simulink model "model"  (R2022a)
settings: Solver=VariableStepAuto  StartTime=0.0  StopTime=5  RelTol=1e-3  EnableMultiTasking=on
values from neighbouring files (symbols this model uses):
  Ce = 0.556    [Untitled.m]    (also in liner.m)
  Ki = 5    [Untitled.m]    (also in liner.m = 1)
  Kn = 7.84    [Untitled.m]    (also in liner.m = 29.75)
  Ks = 1    [Untitled.m]    (also in liner.m)
  R = 0.6    [Untitled.m]    (also in liner.m)
  Tl = 0.167    [Untitled.m]    (also in liner.m)
  Tm = 0.282    [Untitled.m]    (also in liner.m)
  Toi = 0.0025    [Untitled.m]
  Ton = 0.1    [Untitled.m]
  Ts = 0.01    [Untitled.m]    (also in liner.m)
undefined symbols (not defined in the file or in its folder): alpha, beta, Id, IdN, taui, taun, Ud, UN, Un, Uoil, Uonl
settings Model: Creator=houtonglei  LastModifiedBy=houtonglei
settings SolverCC: AllowMultiTaskInputOutput=on  ConcurrentTasks=on  AlgebraicLoopSolver=TrustRegion  PositivePriorityOrder=on  AutoInsertRateTranBlk=on
settings DataIOCC: SaveFinalState=on
settings OptimizationCC: UseDivisionForNetSlopeComputation=UseDivisionForReciprocalsOfIntegersOnly  GainParamInheritBuiltInType=on  UseFloatMulNetSlope=on  InheritOutputTypeSmallerThanSingle=on  UseRowMajorAlgorithm=on
settings DebuggingCC: ReadBeforeWriteMsg=DisableAll  WriteAfterWriteMsg=DisableAll  WriteAfterReadMsg=DisableAll
settings ModelReferenceCC: EnableParallelModelReferenceBuilds=on  ParallelModelReferenceMATLABWorkerInit=Load Top Model  ModelReferenceMinAlgLoopOccurrences=on
settings SFSimCC: SFSimEcho=off  CustomCodeUndefinedFunction=UseInterfaceOnly

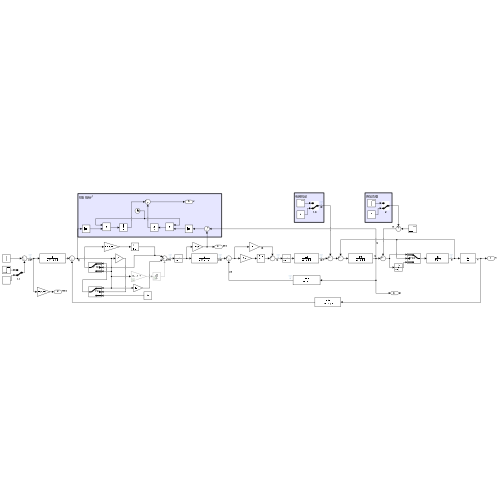
[thumbnail: Simulink's stored preview of the top-level diagram]
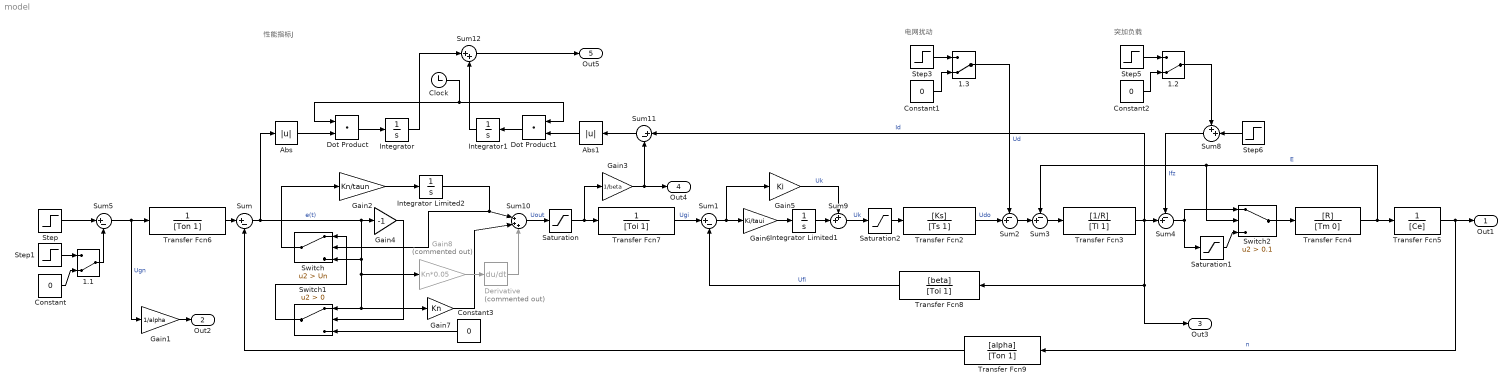
== system model ==
  note: 性能指标J
  note: 突加负载
  note: 电网扰动
  1.1 : ManualSwitch  CurrentSetting=0
  1.2 : ManualSwitch  CurrentSetting=0
  1.3 : ManualSwitch  CurrentSetting=0
  Abs : Abs  SaturateOnIntegerOverflow=off
  Abs1 : Abs  SaturateOnIntegerOverflow=off
  Clock : Clock
  Constant{,1..3} (4 alike) : Constant  Value=0
  Derivative : Derivative  Commented=on
  Dot Product : DotProduct  OutDataTypeStr=Inherit: Inherit via internal rule
  Dot Product1 : DotProduct  OutDataTypeStr=Inherit: Inherit via internal rule
  Gain1 : Gain  Gain=1/alpha
  Gain2 : Gain  Gain=Kn/taun
  Gain3 : Gain  Gain=1/beta
  Gain4 : Gain  Gain=-1
  Gain5 : Gain  Gain=Ki
  Gain6 : Gain  Gain=Ki/taui
  Gain7 : Gain  Gain=Kn
  Gain8 : Gain  Commented=on  Gain=Kn*0.05
  Integrator : Integrator
  Integrator Limited1 : Integrator  LimitOutput=on  UpperSaturationLimit=Uoil  LowerSaturationLimit=-Uoil
  Integrator Limited2 : Integrator  LimitOutput=on  UpperSaturationLimit=Uonl  LowerSaturationLimit=-Uonl
  Integrator1 : Integrator
  Saturation : Saturate  UpperLimit=Uonl  LowerLimit=-Uonl
  Saturation1 : Saturate  UpperLimit=IdN  LowerLimit=0
  Saturation2 : Saturate  UpperLimit=Uoil  LowerLimit=-Uoil
  Step : Step  Time=0  After=Ud  SampleTime=0
  Step1 : Step  After=2  SampleTime=0
  Step3 : Step  After=0.1 * UN  SampleTime=0
  Step5 : Step  After=0.5*IdN  SampleTime=0
  Step6 : Step  Time=0  After=Id  SampleTime=0
  Sum{,1,5,11} (4 alike) : Sum  Inputs=|+-
  Sum10 : Sum  Inputs=|+++
  Sum12 : Sum  Inputs=|++
  Sum2 : Sum  Inputs=-+|
  Sum3 : Sum  Inputs=-+|
  Sum4 : Sum  Inputs=-+|
  Sum8 : Sum  Inputs=++|
  Sum9 : Sum  Inputs=++|
  Switch : Switch  Criteria=u2 > Threshold  Threshold=Un  SaturateOnIntegerOverflow=off  InputSameDT=off
  Switch1 : Switch  Criteria=u2 > Threshold  SaturateOnIntegerOverflow=off  InputSameDT=off
  Switch2 : Switch  Criteria=u2 > Threshold  Threshold=0.1  SaturateOnIntegerOverflow=off  InputSameDT=off
  Transfer Fcn2 : TransferFcn  Numerator=[Ks]  Denominator=[Ts 1]  ContinuousStateAttributes='PWM'
  Transfer Fcn3 : TransferFcn  Numerator=[1/R]  Denominator=[Tl 1]
  Transfer Fcn4 : TransferFcn  Numerator=[R]  Denominator=[Tm 0]
  Transfer Fcn5 : TransferFcn  Denominator=[Ce]
  Transfer Fcn6 : TransferFcn  Denominator=[Ton 1]  ContinuousStateAttributes='ACR'
  Transfer Fcn7 : TransferFcn  Denominator=[Toi 1]  ContinuousStateAttributes='ACR'
  Transfer Fcn8 : TransferFcn  Numerator=[beta]  Denominator=[Toi 1]  ContinuousStateAttributes='ACR'
  Transfer Fcn9 : TransferFcn  Numerator=[alpha]  Denominator=[Ton 1]  ContinuousStateAttributes='ACR'
  Out1 : Outport  SignalName=n
  Out2 : Outport  Port=2  SignalName=nref
  Out3 : Outport  Port=3  SignalName=Id
  Out4 : Outport  Port=4  SignalName=Iref
  Out5 : Outport  Port=5  SignalName=J
  wires:
  Transfer Fcn9/1 -> Sum/2
  Transfer Fcn8/1 -> Sum1/2  "Ufi"
  Clock/1 -> Dot Product/1, Dot Product1/1
  Abs/1 -> Dot Product/2
  Dot Product/1 -> Integrator/1
  Sum3/1 -> Transfer Fcn3/1
  Transfer Fcn3/1 -> Sum4/2, Out3/1, Transfer Fcn8/1, Sum11/1  "Id"
  Step/1 -> Sum5/1
  Step1/1 -> 1.1/1
  Constant/1 -> 1.1/2
  Constant1/1 -> 1.3/2
  Step3/1 -> 1.3/1
  Constant2/1 -> 1.2/2
  Step5/1 -> 1.2/1
  1.2/1 -> Sum8/1
  Step6/1 -> Sum8/2
  Transfer Fcn6/1 -> Sum/1
  Sum5/1 -> Transfer Fcn6/1, Gain1/1  "Ugn"
  Transfer Fcn7/1 -> Sum1/1  "Ugi"
  Sum9/1 -> Saturation2/1  "Uk"
  Saturation2/1 -> Transfer Fcn2/1
  Saturation/1 -> Transfer Fcn7/1, Gain3/1
  Saturation1/1 -> Switch2/3
  Sum4/1 -> Switch2/1, Saturation1/1
  Switch2/1 -> Transfer Fcn4/1
  Transfer Fcn4/1 -> Transfer Fcn5/1, Sum3/1, Switch2/2  "E"
  Transfer Fcn5/1 -> Out1/1, Transfer Fcn9/1  "n"
  Gain6/1 -> Integrator Limited1/1
  Gain5/1 -> Sum9/1  "Uk"
  Integrator Limited1/1 -> Sum9/2
  Sum1/1 -> Gain5/1, Gain6/1
  Sum8/1 -> Sum4/1  "Ifz"
  Transfer Fcn2/1 -> Sum2/2  "Udo"
  Sum2/1 -> Sum3/2
  1.3/1 -> Sum2/1  "Ud"
  1.1/1 -> Sum5/2
  Gain1/1 -> Out2/1
  Gain3/1 -> Out4/1, Sum11/2
  Switch1/1 -> Switch/1
  Switch/1 -> Gain2/1
  Integrator Limited2/1 -> Sum10/1, Switch/2
  Gain7/1 -> Sum10/2
  Constant3/1 -> Switch1/3
  Sum/1 -> Gain7/1, Switch1/1, Gain8/1, Switch/3, Gain4/1, Abs/1  "e(t)"
  Gain4/1 -> Switch1/2
  Gain8/1 -> Derivative/1
  Gain2/1 -> Integrator Limited2/1
  Derivative/1 -> Sum10/3
  Sum10/1 -> Saturation/1  "Uout"
  Dot Product1/1 -> Integrator1/1
  Integrator1/1 -> Sum12/2
  Integrator/1 -> Sum12/1
  Sum12/1 -> Out5/1
  Sum11/1 -> Abs1/1
  Abs1/1 -> Dot Product1/2
